simulink model "pervichNsignal"  (Simulink 8.7)
settings: Solver=ode45  StartTime=0.0  StopTime=0.2  MaxStep=1e-5  RelTol=1e-3
settings Model: Creator=1  LastModifiedBy=blackjets
settings DebuggingCC: UnderspecifiedInitializationDetection=Simplified  MergeDetectMultiDrivingBlocksExec=error

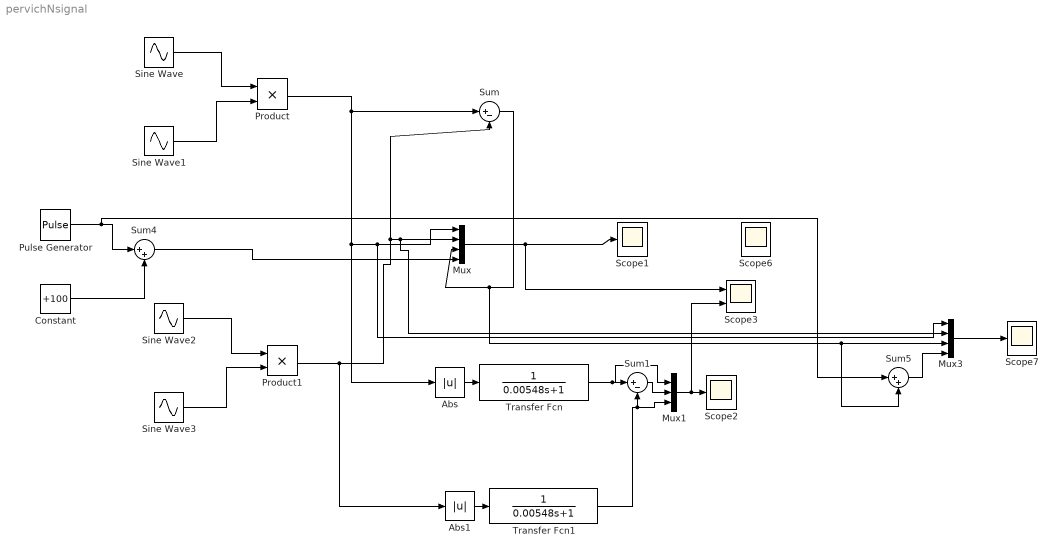
== system pervichNsignal ==
  Abs : Abs
  Abs1 : Abs
  Constant : Constant  Value=+100
  Mux : Mux
  Mux1 : Mux  Inputs=3
  Mux3 : Mux
  Product : Product
  Product1 : Product
  Pulse Generator : DiscretePulseGenerator  PulseType=Time based  Amplitude=200  Period=2*pi/10000  PhaseDelay=((2*pi/10000)/360)*90
  Scope{1..2,6..7} (4 alike) : Scope
  Scope3 : Scope  NumInputPorts=2
  Sine Wave : Sin  Amplitude=10  Frequency=10000  SampleTime=0
  Sine Wave1 : Sin  Amplitude=2  Bias=10  Frequency=1000  SampleTime=0
  Sine Wave2 : Sin  Amplitude=10  Frequency=10000  Phase=pi/180*10  SampleTime=0
  Sine Wave3 : Sin  Amplitude=2  Bias=10  Frequency=1000  Phase=2*pi/2  SampleTime=0
  Sum : Sum  Inputs=|+-
  Sum1 : Sum  Inputs=|+-
  Sum4 : Sum  Inputs=|++
  Sum5 : Sum  Inputs=|++
  Transfer Fcn : TransferFcn  Denominator=[0.00548 1]
  Transfer Fcn1 : TransferFcn  Denominator=[0.00548 1]
  wires:
  Sine Wave/1 -> Product/1
  Sine Wave1/1 -> Product/2
  Sine Wave2/1 -> Product1/1
  Sine Wave3/1 -> Product1/2
  Product/1 -> Abs/1, Mux3/1, Mux/1, Sum/1
  Mux/1 -> Scope1/1, Scope3/1
  Sum/1 -> Sum5/2, Mux3/3, Mux/3
  Transfer Fcn/1 -> Mux1/1, Sum1/1
  Mux1/1 -> Scope3/2, Scope2/1
  Abs/1 -> Transfer Fcn/1
  Product1/1 -> Abs1/1, Sum/2, Mux3/2, Mux/2
  Transfer Fcn1/1 -> Mux1/3, Sum1/2
  Abs1/1 -> Transfer Fcn1/1
  Sum1/1 -> Mux1/2
  Pulse Generator/1 -> Sum5/1, Sum4/1
  Constant/1 -> Sum4/2
  Sum4/1 -> Mux/4
  Sum5/1 -> Mux3/4
  Mux3/1 -> Scope7/1
